simulink model "problem3"  (R2020b)
settings: Solver=VariableStepAuto  StartTime=0.0  StopTime=10.0  MaxStep=0.0001  RelTol=1e-3
settings Model: Creator=Admin  LastModifiedBy=Admin

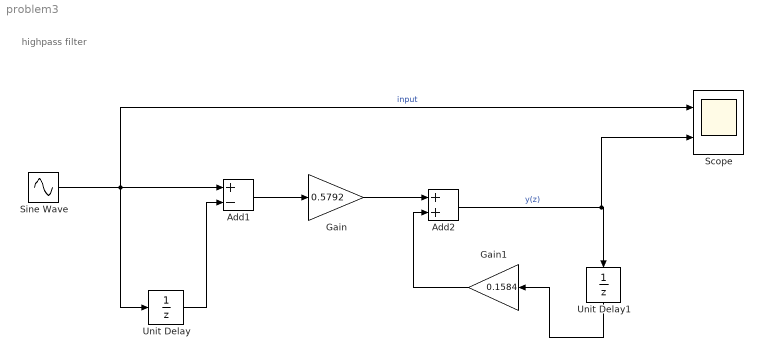
== system problem3 ==
  note: highpass filter
  Add1 : Sum  Inputs=+-
  Add2 : Sum
  Gain : Gain  Gain=0.5792
  Gain1 : Gain  Gain=0.1584
  Scope : Scope  NumInputPorts=2
  Sine Wave : Sin  Frequency=1500  SampleTime=0
  Unit Delay : UnitDelay  SampleTime=-1  HasFrameUpgradeWarning=on
  Unit Delay1 : UnitDelay  SampleTime=-1  HasFrameUpgradeWarning=on
  wires:
  Unit Delay1/1 -> Gain1/1
  Add1/1 -> Gain/1
  Sine Wave/1 -> Unit Delay/1, Scope/1, Add1/1  "input"
  Gain1/1 -> Add2/2
  Add2/1 -> Scope/2, Unit Delay1/1  "y(z)"
  Gain/1 -> Add2/1
  Unit Delay/1 -> Add1/2
